simulink model "Basic_DMT"  (R2014b)
settings: Solver=FixedStepDiscrete  SolverMode=SingleTasking  StartTime=0.0  StopTime=25e-6-14e-9*24  RelTol=1e-3
PreLoadFcn:
  | userName = getenv('UserName');
  | 
  | if strcmp(userName,'Tim')
  | cd C:\Users\Tim\Documents\GitHub\MA_1\Basic_DMT
  | else
  | cd C:\Users\Tim-UML\Documents\GitHub\MA_1\Basic_DMT
  | end
InitFcn:
  | userName = getenv('UserName');
  | 
  | if strcmp(userName,'Tim')
  | cd C:\Users\Tim\Documents\GitHub\MA_1\Basic_DMT
  | else
  | cd C:\Users\Tim-UML\Documents\GitHub\MA_1\Basic_DMT
  | end
values from neighbouring files (symbols this model uses):
  a0 = 0.21194908595403703    (= 0.211949085954)    [initScript.m]
  a1 = 0.576101828091926    (= 0.576101828092)    [initScript.m]
  a2 = a0    (= 0.211949085954)    [initScript.m]
  beta = 1    [initScript.m]
  bitPerSymb = 4    [initScript.m]
  chanDownFact = Tchan/SystemPeriod    [initScript.m]
  fftLen = 16    [initScript.m]
  fftLenActive = fftLenDMT    (= 32)    [initScript.m]
  fftLenDMT = 2*fftLen    (= 32)    [initScript.m]
  GI_Active = GI_LenDMT    (= 0)    [initScript.m]
  GI_Len = 0    [initScript.m]
  GI_LenDMT = 0    [initScript.m]
  M = log2(fftLen)    [initScript.m]
  sysgenSystemPeriod = 4e-9    (= 4e-09)    [initScript.m]
  SystemPeriod = 4e-9    (= 4e-09)    [initScript.m]
  upsampleFactor = 1    [initScript.m]
  usedSubCar = 14    [initScript.m]
undefined symbols (not defined in the file or in its folder): bitCount, get, modu_mode, Tb, Ts
libraries: xbsIndex_r4 x822, commdigbbndam3 x59, simulink x42, dspsigops x7, commrandsrc2 x6, dspbuff3 x4, dspxfrm3 x3, dspswit3 x2, commseqgen2 x1, dsparch4 x1, commutil2 x1, dspsnks4 x1
(part 1 of 10)
settings Model: Creator=Tim-UML  LastModifiedBy=Tim-UML
settings DebuggingCC: AssertControl=DisableAll
settings HardwareCC: ProdBitPerLong=64  ProdBitPerPointer=64  ProdWordSize=64  ProdHWDeviceType=Generic->64-bit Embedded Processor (LP64)  TargetHWDeviceType=32-bit Generic

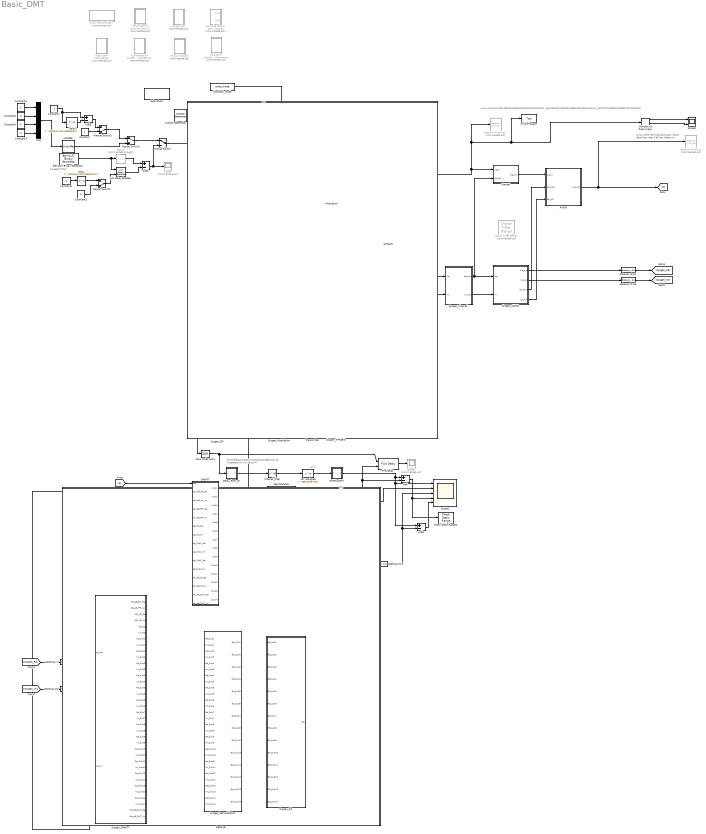
== system Basic_DMT ==
  note: www.marcuswinter.de%2Fmedia%2FOFDM%2FCP%252520spectra.png&imgrefurl=http%3A%2F%2Fwww.marcuswinter.de%2Farchives%2F884&h=684&w=400&tbnid=4qO6ZL-0OhDcYM%3A&docid=MqEDPGI0eCEqiM&ei=dVTEVrCJIeWP6ATR9aGoBQ&tbm=isch&iact=rc&uact=3&dur=395&page=1&start=0&ndsp=36&ved=0ahUKEwjwl_qN1P7KAhXlB5oKHdF6CFUQrQMIIDAA
  note: 477
  note: 1/1.5e8==Ts/3
  note: Umso höher die Modulationsart, desto
      |  deutlicher über 0 dB das Spektrum
  note: 32 singletasking 64 multitasking 256-QAM
      | 16 singletaskink mit 16-QAM
  " System Generator" : xbsIndex_r4/ System Generator  Tag=genX  xilinxfamily=zynq  part=xc7z020  speed=-1  package=clg400  synthesis_tool=Vivado  clock_wrapper=Clock Enables  directory=./netlist  proj_type=Vivado  Synth_file=Vivado Synthesis Defaults  Impl_file=Vivado Implementation Defaults  testbench=off  simulink_period=sysgenSystemPeriod  sysclk_period=1000/250  dcm_input_clock_period=10  incr_netlist=off  trim_vbits=Everywhere in SubSystem  dbl_ovrd=According to Block Masks  core_generation=According to Block Masks  run_coregen=off  deprecated_control=off  eval_field=0  block_type=sysgen
  16-QAM Sysgen : Subsystem  Commented=on
  AWGN : Subsystem  Variant=on
  Add{,1..3} (4 alike) : Sum  Inputs=+-
  Bernoulli Binary Generator : commrandsrc2/Bernoulli Binary Generator  P=0.5  seed=1604198  Ts=Tb  frameBased=off  sampPerFrame=1  orient=off  outDataType=boolean
      settings: AttributesFormatString=|
      | Sample Time= %<Ts>
      | Prob zero=%<P>
  Channel : Subsystem  Variant=on
  Channel_filter : Delay  DelayLength=56  InitialCondition=0
  Check Static Range2 : simulink/Model Verification/Check  Static Range  Description=0 <= u <= 0  max=0  max_included=on  min=0  min_included=on  enabled=off  stopWhenAssertionFail=on  export=off  icon=graphic
  Combination of Sysgen S/P and 16QAM : Subsystem  Commented=on
  Complex to Real-Imag1 : ComplexToRealImag
  Constant : Constant  SampleTime=Tb
  Constant1 : Constant  SampleTime=Tb
  Constant2 : Constant  Value=0  SampleTime=Tb
  Constant3 : Constant  Value=0  SampleTime=Tb*4
  Constant4 : Constant  SampleTime=Tb*4
  Constant5 : Constant  Value=0  SampleTime=Tb*4
  Constant6 : Constant  Value=0  SampleTime=Tb*4
  Constant7 : Constant  SampleTime=Tb
  Constant_mode : Constant  Value=modu_mode  OutDataTypeStr=single
  Delay : Delay  DelayLength=bitPerSymb*usedSubCar-1  InitialCondition=0
  Delay1 : Delay  Commented=through  DelayLength=1  InitialCondition=0
  Delay3 : Delay  DelayLength=bitPerSymb*usedSubCar  InitialCondition=0
  Delay_Rem_GI : Subsystem  Variant=on
  Demodulation : Subsystem
  Digital Filter Design : dsparch4/Digital Filter Design  Commented=on  mwdsp_browser_bugfix_var=off
  Examine Slice Block : Subsystem  Commented=on
  Find Delay : commutil2/Find Delay  corrLength=1000  chgSigOP=off  stopUpdate=off  numConstDelay=3
  Gateway In : xbsIndex_r4/Gateway In  gui_display_data_type=Fixed-point  arith_type="Signed  (2's comp)"  n_bits=bitCount+log2(fftLen)+1  bin_pt=fracLen  preci_type=Single  exp_width=8  frac_width=24  rows=1  columns=1  quantization="Round  (unbiased: +/- Inf)"  overflow=Saturate  period=Ts*M*usedSubCar/(fftLenActive+GI_Active)  UseAsADC=off  ADCChannel='1'  interface=None  automatic_assignment=on  address_offset=hex2dec('00')  intf_description=''  timing_constraint=None  locs_specified=off  LOCs={}  io_standard={}  inherit_from_input=off  hdl_port=on  dbl_ovrd=off  block_type=gatewayin
  Gateway In1 : xbsIndex_r4/Gateway In  gui_display_data_type=Fixed-point  arith_type="Signed  (2's comp)"  n_bits=bitCount+log2(fftLen)+1  bin_pt=fracLen  preci_type=Single  exp_width=8  frac_width=24  rows=1  columns=1  quantization="Round  (unbiased: +/- Inf)"  overflow=Saturate  period=Ts*M*usedSubCar/(fftLenActive+GI_Active)  UseAsADC=off  ADCChannel='1'  interface=None  automatic_assignment=on  address_offset=hex2dec('00')  intf_description=''  timing_constraint=None  locs_specified=off  LOCs={}  io_standard={}  inherit_from_input=off  hdl_port=on  dbl_ovrd=off  block_type=gatewayin
  Gateway Out : xbsIndex_r4/Gateway Out  inherit_from_input=on  hdl_port=on  rows=1  columns=1  UseAsDAC=off  DACChannel='1'  interface=None  automatic_assignment=on  address_offset=hex2dec('00')  intf_description=''  timing_constraint=None  locs_specified=off  LOCs={}  io_standard={}  block_type=gatewayout
  Gateway Out4 : xbsIndex_r4/Gateway Out  inherit_from_input=on  hdl_port=on  rows=1  columns=1  UseAsDAC=off  DACChannel='1'  interface=None  automatic_assignment=on  address_offset=hex2dec('00')  intf_description=''  timing_constraint=None  locs_specified=off  LOCs={}  io_standard={}  block_type=gatewayout
  Gateway Out5 : xbsIndex_r4/Gateway Out  inherit_from_input=on  hdl_port=on  rows=1  columns=1  UseAsDAC=off  DACChannel='1'  interface=None  automatic_assignment=on  address_offset=hex2dec('00')  intf_description=''  timing_constraint=None  locs_specified=off  LOCs={}  io_standard={}  block_type=gatewayout
  IFFTaPIS : Subsystem
  Manual Switch : ManualSwitch
  Manual Switch1 : ManualSwitch
  Manual Switch2 : ManualSwitch  CurrentSetting=0
  Manual Switch3 : ManualSwitch  CurrentSetting=0
  Modulation : Subsystem
  Mux : Mux
  OFDMorDMT : Subsystem  Variant=on
  "PIS " : Subsystem
  Receiver : Subsystem
  "SIP " : Subsystem  RequirementInfo="{}  %GIDa_16a870dd_20fa_4000_a28f_04c7e291452f"
  SIPaFFT : Subsystem
  Scope : Scope  Commented=on
      settings: SaveName=ScopeData65
  Scope1 : Scope  Commented=on
      settings: YMin=-1  YMax=1  SaveName=ScopeData6
  Scope2 : Scope  NumInputPorts=5
      settings: YMin=0~0~0~-1~-1  YMax=1~1~1~1~1  SaveName=ScopeData2
  Scope3 : Scope  NumInputPorts=2
      settings: YMin=-10~-8  YMax=8~8  SaveName=ScopeData30
  Spectrum Analyzer : SpectrumAnalyzer  Commented=on
  Spectrum Analyzer1 : SpectrumAnalyzer  Commented=on
  Subsystem : Subsystem  mask(Model Parameters){upsample=No, dmtOfdm=OFDM, guardInterval=No, AWGN=No, channel=No, equalizer=No, SampleTime=20e-9, BitTime=20e-9, modu_mode=0, radio_precision=double, bitCount=16, fracLen=13, impulseResponse=No}
      mask prompts: upsample "Enable Upsampling"; dmtOfdm "Select FFT Inputorder"; guardInterval "Guard Interval"; SampleTime "Sample Time [s]"; BitTime "Bit Time"; modu_mode "Modulation Mode"; radio_precision "Select Precision"; bitCount "Bit Count"; fracLen "Fraction Length"; impulseResponse "Measure Impulse Response"
      mask init:
      | initScript
      mask TypeOptions upsample: No | Yes
      mask TypeOptions dmtOfdm: OFDM | DMT
      mask TypeOptions guardInterval: No | Yes
      mask TypeOptions AWGN: No | Yes
      mask TypeOptions channel: No | Yes
      mask TypeOptions equalizer: No | Yes
      mask TypeOptions radio_precision: double | fixpoint
      mask TypeOptions impulseResponse: No | Yes
      mask DialogControl Container3 Prompt: Only for Fixpoint
      mask Display: disp('Edit Model\n Parameters')
  Sysgen S/P1 : Subsystem  Commented=on
  Sysgen_AWGN : Subsystem  Variant=on
  Sysgen_Channel : Subsystem  Variant=on
  Sysgen_Demodulation : Subsystem
  Sysgen_IFFTaPIS : Subsystem
  Sysgen_Modulation : Subsystem
  Sysgen_PIS : Subsystem
  Sysgen_SIP : Subsystem
  Sysgen_SIPaFFT : Subsystem
  Testsystem Channelfilter : Subsystem  Commented=on
  Testsystem to examine Demux : Subsystem  Commented=on
  To Workspace : ToWorkspace  VariableName=Test  SampleTime=-1
      settings: Save2DSignal=2-D array (concatenate along first dimension)
  Total Bits / Subchannel Information : Subsystem  Commented=on
  Transmitter : Subsystem
  Unbuffer : Unbuffer  SampleBasedProcessing=Same as frame based
  Unit Delay Enabled : simulink/Additional Math & Discrete/Additional Discrete/Unit Delay Enabled  vinit=0.0  tsamp=-1
  Versuche DEMUX verm. löschen : Subsystem  Commented=on
  Zero-Order Hold : ZeroOrderHold  SampleTime=Ts
  not_assigned : Delay  DelayLength=589-16*8+8*2  InitialCondition=0
  wires:
  Manual Switch/1 -> "SIP "/1(S1), Zero-Order Hold/1, Sysgen_SIP/1(Inp)
  Add/1 -> Scope2/4, Check Static Range2/1
  "PIS "/1(Out) -> Find Delay/2, Add/2, Scope2/2
  Constant_mode/1 -> Demodulation/15(mode), Modulation/15(mode)
  Demodulation/1(Sub1_out) -> "PIS "/1(Sub1)
  Demodulation/2(Sub2_out) -> "PIS "/2(Sub2)
  Modulation/2(Sub2_out) -> IFFTaPIS/2(Sub2)
  SIPaFFT/1(Sub1) -> Demodulation/1(Sub1)
  SIPaFFT/2(Sub2) -> Demodulation/2(Sub2)
  Find Delay/1 -> Scope1/1
  Bernoulli Binary Generator/1 -> Unit Delay Enabled/1, Delay1/1
  Sysgen_Modulation/1(Re_Sub1) -> Modulation/16(db_sub1_re), Sysgen_IFFTaPIS/1(Re_Sub1)
  Modulation/1(Sub1_out) -> IFFTaPIS/1(Sub1)
  "SIP "/2(Sub2) -> Modulation/2(Sub2)
  "SIP "/1(Sub1) -> Modulation/1(Sub1)
  Sysgen_SIP/2(Sub2) -> "SIP "/3(Debug2), Sysgen_Modulation/2(Sub2)
  Sysgen_SIP/1(Sub1) -> "SIP "/2(Debug1), Sysgen_Modulation/1(Sub1)
  Sysgen_IFFTaPIS/1(Re) -> IFFTaPIS/15(db1_aft_GI_Re), Sysgen_Channel/1(Re)
  Gateway Out4/1 -> [Sysgen_Re]
  Gateway Out5/1 -> [Sysgen_Im]
  [A] -> SIPaFFT/1(sig)
  [Sysgen_Re] -> Gateway In/1
  [Sysgen_Im] -> Gateway In1/1
  Gateway In/1 -> Sysgen_SIPaFFT/1(sg_Re), SIPaFFT/2(db_bef_GI_Re)
  Gateway In1/1 -> Sysgen_SIPaFFT/2(sg_Im), SIPaFFT/3(db_bef_GI_Im)
  Sysgen_SIPaFFT/1(db_aft_FFT_Re) -> SIPaFFT/4(db_aft_FFT_Re)
  Sysgen_Demodulation/1(Bit_Sub1) -> Sysgen_PIS/1(Bit_Sub1), Demodulation/16(sg_Sub1_Bit)
  Sysgen_Demodulation/2(Bit_Sub2) -> Sysgen_PIS/2(Bit_Sub2), Demodulation/17(sg_Sub2_Bit)
  Gateway Out/1 -> Scope2/3, Add1/2
  Add1/1 -> Scope2/5
  Sysgen_PIS/1(Bit) -> Gateway Out/1, "PIS "/15(sg_Bit)
  "SIP "/3(Sub3) -> Modulation/3(Sub3)
  "SIP "/4(Sub4) -> Modulation/4(Sub4)
  "SIP "/5(Sub5) -> Modulation/5(Sub5)
  "SIP "/6(Sub6) -> Modulation/6(Sub6)
  "SIP "/7(Sub7) -> Modulation/7(Sub7)
  "SIP "/8(Sub8) -> Modulation/8(Sub8)
  "SIP "/9(Sub9) -> Modulation/9(Sub9)
  "SIP "/10(Sub10) -> Modulation/10(Sub10)
  "SIP "/11(Sub11) -> Modulation/11(Sub11)
  Modulation/3(Sub3_out) -> IFFTaPIS/3(Sub3)
  Modulation/4(Sub4_out) -> IFFTaPIS/4(Sub4)
  Modulation/5(Sub5_out) -> IFFTaPIS/5(Sub5)
  Modulation/6(Sub6_out) -> IFFTaPIS/6(Sub6)
  Modulation/7(Sub7_out) -> IFFTaPIS/7(Sub7)
  Modulation/8(Sub8_out) -> IFFTaPIS/8(Sub8)
  Modulation/9(Sub9_out) -> IFFTaPIS/9(Sub9)
  Modulation/10(Sub10_out) -> IFFTaPIS/10(Sub10)
  Modulation/11(Sub11_out) -> IFFTaPIS/11(Sub11)
  Sysgen_IFFTaPIS/3(Db_aft_frame_Re) -> IFFTaPIS/17(db_aft_frame_Re)
  Sysgen_IFFTaPIS/4(Db_aft_frame_Im) -> IFFTaPIS/18(db_aft_frame_Im)
  Sysgen_IFFTaPIS/5(Db_aft_FFT_Re) -> IFFTaPIS/19(db_FFT_Re)
  Sysgen_IFFTaPIS/6(Db_aft_FFT_Im) -> IFFTaPIS/20(db_FFT_Im)
  SIPaFFT/3(Sub3) -> Demodulation/3(Sub3)
  SIPaFFT/4(Sub4) -> Demodulation/4(Sub4)
  SIPaFFT/5(Sub5) -> Demodulation/5(Sub5)
  SIPaFFT/6(Sub6) -> Demodulation/6(Sub6)
  SIPaFFT/7(Sub7) -> Demodulation/7(Sub7)
  SIPaFFT/8(Sub8) -> Demodulation/8(Sub8)
  SIPaFFT/9(Sub9) -> Demodulation/9(Sub9)
  SIPaFFT/10(Sub10) -> Demodulation/10(Sub10)
  SIPaFFT/11(Sub11) -> Demodulation/11(Sub11)
  Demodulation/3(Sub3_out) -> "PIS "/3(Sub3)
  Demodulation/4(Sub4_out) -> "PIS "/4(Sub4)
  Demodulation/5(Sub5_out) -> "PIS "/5(Sub5)
  Demodulation/6(Sub6_out) -> "PIS "/6(Sub6)
  Demodulation/7(Sub7_out) -> "PIS "/7(Sub7)
  Demodulation/8(Sub8_out) -> "PIS "/8(Sub8)
  Demodulation/9(Sub9_out) -> "PIS "/9(Sub9)
  Demodulation/10(Sub10_out) -> "PIS "/10(Sub10)
  Demodulation/11(Sub11_out) -> "PIS "/11(Sub11)
  Modulation/12(Sub12_out) -> IFFTaPIS/12(Sub12)
  Modulation/13(Sub13_out) -> IFFTaPIS/13(Sub13)
  Modulation/14(Sub14_out) -> IFFTaPIS/14(Sub14)
  SIPaFFT/14(Sub14) -> Demodulation/14(Sub14)
  SIPaFFT/13(Sub13) -> Demodulation/13(Sub13)
  SIPaFFT/12(Sub12) -> Demodulation/12(Sub12)
  Demodulation/13(Sub13_out) -> "PIS "/13(Sub13)
  Demodulation/14(Sub14_out) -> "PIS "/14(Sub14)
  Demodulation/12(Sub12_out) -> "PIS "/12(Sub12)
  "SIP "/12(Sub12) -> Modulation/12(Sub12)
  "SIP "/13(Sub13) -> Modulation/13(Sub13)
  "SIP "/14(Sub14) -> Modulation/14(Sub14)
  OFDMorDMT/1(Out1) -> Add1/1, Scope2/1, Add/1
  Sysgen_SIP/3(Sub3) -> Sysgen_Modulation/3(Sub3)
  Sysgen_SIP/4(Sub4) -> Sysgen_Modulation/4(Sub4)
  Sysgen_SIP/5(Sub5) -> Sysgen_Modulation/5(Sub5)
  Sysgen_SIP/6(Sub6) -> Sysgen_Modulation/6(Sub6)
  Sysgen_SIP/7(Sub7) -> Sysgen_Modulation/7(Sub7)
  Sysgen_SIP/8(Sub8) -> Sysgen_Modulation/8(Sub8)
  Sysgen_SIP/9(Sub9) -> Sysgen_Modulation/9(Sub9)
  Sysgen_SIP/10(Sub10) -> Sysgen_Modulation/10(Sub10)
  Sysgen_SIP/11(Sub11) -> Sysgen_Modulation/11(Sub11)
  Sysgen_SIP/12(Sub12) -> Sysgen_Modulation/12(Sub12)
  Sysgen_SIP/13(Sub13) -> Sysgen_Modulation/13(Sub13)
  Sysgen_SIP/14(Sub14) -> Sysgen_Modulation/14(Sub14)
  Sysgen_Modulation/2(Im_Sub1) -> Modulation/17(db_sub1_im), Sysgen_IFFTaPIS/2(Im_Sub1)
  Sysgen_Modulation/3(Re_Sub2) -> Modulation/18(db_sub2_re), Sysgen_IFFTaPIS/3(Re_Sub2)
  Sysgen_Modulation/4(Im_Sub2) -> Modulation/19(db_sub2_im), Sysgen_IFFTaPIS/4(Im_Sub2)
  Sysgen_Modulation/5(Re_Sub3) -> Sysgen_IFFTaPIS/5(Re_Sub3)
  Sysgen_Modulation/6(Im_Sub3) -> Sysgen_IFFTaPIS/6(Im_Sub3)
  Sysgen_Modulation/7(Re_Sub4) -> Sysgen_IFFTaPIS/7(Re_Sub4)
  Sysgen_Modulation/8(Im_Sub4) -> Sysgen_IFFTaPIS/8(Im_Sub4)
  Sysgen_Modulation/9(Re_Sub5) -> Sysgen_IFFTaPIS/9(Re_Sub5)
  Sysgen_Modulation/10(Im_Sub5) -> Sysgen_IFFTaPIS/10(Im_Sub5)
  Sysgen_Modulation/11(Re_Sub6) -> Sysgen_IFFTaPIS/11(Re_Sub6)
  Sysgen_Modulation/12(Im_Sub6) -> Sysgen_IFFTaPIS/12(Im_Sub6)
  Sysgen_Modulation/13(Re_Sub7) -> Sysgen_IFFTaPIS/13(Re_Sub7)
  Sysgen_Modulation/14(Im_Sub7) -> Sysgen_IFFTaPIS/14(Im_Sub7)
  Sysgen_Modulation/15(Re_Sub8) -> Sysgen_IFFTaPIS/15(Re_Sub8)
  Sysgen_Modulation/16(Im_Sub8) -> Sysgen_IFFTaPIS/16(Im_Sub8)
  Sysgen_Modulation/17(Re_Sub9) -> Sysgen_IFFTaPIS/17(Re_Sub9)
  Sysgen_Modulation/18(Im_Sub9) -> Sysgen_IFFTaPIS/18(Im_Sub9)
  Sysgen_Modulation/19(Re_Sub10) -> Sysgen_IFFTaPIS/19(Re_Sub10)
  Sysgen_Modulation/20(Im_Sub10) -> Sysgen_IFFTaPIS/20(Im_Sub10)
  Sysgen_Modulation/21(Re_Sub11) -> Sysgen_IFFTaPIS/21(Re_Sub11)
  Sysgen_Modulation/22(Im_Sub11) -> Sysgen_IFFTaPIS/22(Im_Sub11)
  Sysgen_Modulation/23(Re_Sub12) -> Sysgen_IFFTaPIS/23(Re_Sub12)
  Sysgen_Modulation/24(Im_Sub12) -> Sysgen_IFFTaPIS/24(Im_Sub12)
  Sysgen_Modulation/25(Re_Sub13) -> Sysgen_IFFTaPIS/25(Re_Sub13)
  Sysgen_Modulation/26(Im_Sub13) -> Sysgen_IFFTaPIS/26(Im_Sub13)
  Sysgen_Modulation/27(Re_Sub14) -> Sysgen_IFFTaPIS/27(Re_Sub14)
  Sysgen_Modulation/28(Im_Sub14) -> Sysgen_IFFTaPIS/28(Im_Sub14)
  not_assigned/1 -> OFDMorDMT/1(In1)
  Sysgen_SIPaFFT/34(Im_Sub14) -> Sysgen_Demodulation/28(Im_Sub14)
  Sysgen_SIPaFFT/33(Re_Sub14) -> Sysgen_Demodulation/27(Re_Sub14)
  Sysgen_SIPaFFT/32(Im_Sub13) -> Sysgen_Demodulation/26(Im_Sub13)
  Sysgen_SIPaFFT/31(Re_Sub13) -> Sysgen_Demodulation/25(Re_Sub13)
  Sysgen_SIPaFFT/30(Im_Sub12) -> Sysgen_Demodulation/24(Im_Sub12)
  Sysgen_SIPaFFT/29(Re_Sub12) -> Sysgen_Demodulation/23(Re_Sub12)
  Sysgen_SIPaFFT/28(Im_Sub11) -> Sysgen_Demodulation/22(Im_Sub11)
  Sysgen_SIPaFFT/27(Re_Sub11) -> Sysgen_Demodulation/21(Re_Sub11)
  Sysgen_SIPaFFT/26(Im_Sub10) -> Sysgen_Demodulation/20(Im_Sub10)
  Sysgen_SIPaFFT/25(Re_Sub10) -> Sysgen_Demodulation/19(Re_Sub10)
  Sysgen_SIPaFFT/24(Im_Sub9) -> Sysgen_Demodulation/18(Im_Sub9)
  Sysgen_SIPaFFT/23(Re_Sub9) -> Sysgen_Demodulation/17(Re_Sub9)
  Sysgen_SIPaFFT/22(Im_Sub8) -> Sysgen_Demodulation/16(Im_Sub8)
  Sysgen_SIPaFFT/21(Re_Sub8) -> Sysgen_Demodulation/15(Re_Sub8)
  Sysgen_SIPaFFT/20(Im_Sub7) -> Sysgen_Demodulation/14(Im_Sub7)
  Sysgen_SIPaFFT/19(Re_Sub7) -> Sysgen_Demodulation/13(Re_Sub7)
  Sysgen_SIPaFFT/18(Im_Sub6) -> Sysgen_Demodulation/12(Im_Sub6)
  Sysgen_SIPaFFT/17(Re_Sub6) -> Sysgen_Demodulation/11(Re_Sub6)
  Sysgen_SIPaFFT/16(Im_Sub5) -> Sysgen_Demodulation/10(Im_Sub5)
  Sysgen_SIPaFFT/15(Re_Sub5) -> Sysgen_Demodulation/9(Re_Sub5)
  Sysgen_SIPaFFT/14(Im_Sub4) -> Sysgen_Demodulation/8(Im_Sub4)
  Sysgen_SIPaFFT/11(Re_Sub3) -> Sysgen_Demodulation/5(Re_Sub3)
  Sysgen_SIPaFFT/12(Im_Sub3) -> Sysgen_Demodulation/6(Im_Sub3)
  Sysgen_SIPaFFT/13(Re_Sub4) -> Sysgen_Demodulation/7(Re_Sub4)
  Sysgen_SIPaFFT/10(Im_Sub2) -> SIPaFFT/11(sg_Sub2_Im), Sysgen_Demodulation/4(Im_Sub2)
  Sysgen_SIPaFFT/9(Re_Sub2) -> SIPaFFT/10(sg_Sub2_Re), Sysgen_Demodulation/3(Re_Sub2)
  Sysgen_SIPaFFT/8(Im_Sub1) -> SIPaFFT/9(sg_Sub1_Im), Sysgen_Demodulation/2(Im_Sub1)
  Sysgen_SIPaFFT/7(Re_Sub1) -> SIPaFFT/8(sg_Sub1_Re), Sysgen_Demodulation/1(Re_Sub1)
  Sysgen_SIPaFFT/2(db_aft_FFT_Im) -> SIPaFFT/5(db_aft_FFT_Im)
  Sysgen_SIPaFFT/3(db2_GI_Re) -> SIPaFFT/12(db_aft_GI_Re)
  Sysgen_SIPaFFT/4(db2_GI_Im) -> SIPaFFT/13(db_aft_GI_Im)
  Sysgen_SIPaFFT/5(Re_DC) -> SIPaFFT/6(sg_DC_Re)
  Sysgen_SIPaFFT/6(Im_DC) -> SIPaFFT/7(sg_DC_Im)
  Sysgen_Demodulation/3(Bit_Sub3) -> Sysgen_PIS/3(Bit_Sub3)
  Sysgen_Demodulation/4(Bit_Sub4) -> Sysgen_PIS/4(Bit_Sub4)
  Sysgen_Demodulation/5(Bit_Sub5) -> Sysgen_PIS/5(Bit_Sub5)
  Sysgen_Demodulation/6(Bit_Sub6) -> Sysgen_PIS/6(Bit_Sub6)
  Sysgen_Demodulation/7(Bit_Sub7) -> Sysgen_PIS/7(Bit_Sub7)
  Sysgen_Demodulation/8(Bit_Sub8) -> Sysgen_PIS/8(Bit_Sub8)
  Sysgen_Demodulation/9(Bit_Sub9) -> Sysgen_PIS/9(Bit_Sub9)
  Sysgen_Demodulation/10(Bit_Sub10) -> Sysgen_PIS/10(Bit_Sub10)
  Sysgen_Demodulation/11(Bit_Sub11) -> Sysgen_PIS/11(Bit_Sub11)
  Sysgen_Demodulation/12(Bit_Sub12) -> Sysgen_PIS/12(Bit_Sub12)
  Sysgen_Demodulation/13(Bit_Sub13) -> Sysgen_PIS/13(Bit_Sub13)
  Sysgen_Demodulation/14(Bit_Sub14) -> Sysgen_PIS/14(Bit_Sub14)
  AWGN/1(sig_out) -> [A], Spectrum Analyzer/1
  Complex to Real-Imag1/1 -> Scope3/1
  Constant/1 -> Manual Switch3/2
  Sysgen_AWGN/1(Re_out) -> Gateway Out4/1
  Sysgen_AWGN/2(Im_out) -> Gateway Out5/1
  Sysgen_AWGN/3(db_bool) -> AWGN/2(db_bool)
  Sysgen_AWGN/4(db_full) -> AWGN/3(db_full)
  Sysgen_IFFTaPIS/2(Im) -> IFFTaPIS/16(db1_aft_GI_Im), Sysgen_Channel/2(Im)
  Sysgen_Channel/1(Re_out) -> Channel/2(db_Re), Sysgen_AWGN/1(Re)
  Sysgen_Channel/2(Im_out) -> Sysgen_AWGN/2(Im)
  Channel_filter/1 -> not_assigned/1
  Channel/1(sig_out) -> AWGN/1(sig_in)
  Sysgen_SIPaFFT/35(db_aft_DMT_Re) -> SIPaFFT/14(db_aft_DMT_Re)
  Sysgen_SIPaFFT/36(db_aft_DMT_Im) -> SIPaFFT/15(db_aft_DMT_Im)
  Delay_Rem_GI/1(Out1) -> Channel_filter/1
  Complex to Real-Imag1/2 -> Scope3/2
  Add2/1 -> Manual Switch/2, Scope/1
  Unit Delay Enabled/1 -> Add2/2
  Delay/1 -> Manual Switch2/1
  Constant1/1 -> Delay/1
  Delay1/1 -> Add2/1
  Manual Switch2/1 -> Unit Delay Enabled/2
  Constant2/1 -> Manual Switch2/2
  Zero-Order Hold/1 -> Delay_Rem_GI/1(In1), Find Delay/1
  Constant3/1 -> Mux/4
  Constant4/1 -> Mux/1
  Constant5/1 -> Mux/2
  Constant6/1 -> Mux/3
  Mux/1 -> Unbuffer/1
  Unbuffer/1 -> Manual Switch1/2
  Manual Switch1/1 -> Manual Switch/1
  Manual Switch3/1 -> Manual Switch1/1
  Add3/1 -> Manual Switch3/1
  Delay3/1 -> Add3/2
  Constant7/1 -> Add3/1, Delay3/1
  IFFTaPIS/1(Out1) -> Channel/1(sig_in), To Workspace/1, Complex to Real-Imag1/1, Spectrum Analyzer1/1

== system Basic_DMT/16-QAM Sysgen ==
  16-QAM : Subsystem
  Check Static Range1 : simulink/Model Verification/Check  Static Range  Description=0 <= u <= 0  max=0  max_included=on  min=0  min_included=on  enabled=on  stopWhenAssertionFail=on  export=off  icon=graphic
  Complex to Real-Imag : ComplexToRealImag
  Constellation Diagram : ConstellationDiagram
  Data Type Conversion : DataTypeConversion  OutDataTypeStr=fixdt(0,4,0)
  Delay : Delay  DelayLength=1  InitialCondition=0
  Gateway In : xbsIndex_r4/Gateway In  gui_display_data_type=Fixed-point  arith_type=Unsigned  n_bits=4  bin_pt=0  preci_type=Single  exp_width=8  frac_width=24  rows=1  columns=1  quantization="Round  (unbiased: +/- Inf)"  overflow=Saturate  period=Tb  UseAsADC=off  ADCChannel='1'  interface=None  automatic_assignment=on  address_offset=hex2dec('00')  intf_description=''  timing_constraint=None  locs_specified=off  LOCs={}  io_standard={}  inherit_from_input=off  hdl_port=on  dbl_ovrd=off  block_type=gatewayin
  Gateway Out : xbsIndex_r4/Gateway Out  inherit_from_input=off  hdl_port=off  rows=1  columns=1  UseAsDAC=off  DACChannel='1'  interface=None  automatic_assignment=on  address_offset=hex2dec('00')  intf_description=''  timing_constraint=None  locs_specified=off  LOCs={}  io_standard={}  block_type=gatewayout
  Gateway Out1 : xbsIndex_r4/Gateway Out  inherit_from_input=off  hdl_port=off  rows=1  columns=1  UseAsDAC=off  DACChannel='1'  interface=None  automatic_assignment=on  address_offset=hex2dec('00')  intf_description=''  timing_constraint=None  locs_specified=off  LOCs={}  io_standard={}  block_type=gatewayout
  Random Integer Generator : commrandsrc2/Random Integer Generator  mul=16  seed=375435435  Ts=Tb  frameBased=off  sampPerFrame=1  orient=off  outDataType=uint8
  Real-Imag to Complex : RealImagToComplex
  Rect_QAM_Mod : commdigbbndam3/Rectangular QAM Modulator Baseband  M=16  InType=Integer  Enc=Gray  Mapping=[0:15]  PowType=Min. distance between symbols  MinDist=2  AvgPow=1  PeakPow=1  Ph=0  outDtype=double  outWordLen=16  outUDDataType=sfix(8)  outFracLenMode=User-defined  outFracLen=0
  Scope1 : Scope  NumInputPorts=4
      settings: YMin=-5~-5~-5~-5  YMax=5~5~5~5
  Scope2 : Scope  NumInputPorts=3
      settings: YMin=-5~-5~-5  YMax=5~5~5  SaveName=ScopeData19
  Scope3 : Scope
      settings: SaveName=ScopeData3
  Subtract : Sum  Inputs=+-
  wires:
  Real-Imag to Complex/1 -> Constellation Diagram/1
  Gateway Out/1 -> Scope2/2, Subtract/2, Real-Imag to Complex/1, Scope1/1
  Gateway Out1/1 -> Real-Imag to Complex/2, Scope1/2
  Gateway In/1 -> 16-QAM/1(In1)
  16-QAM/1(Out2) -> Gateway Out/1
  16-QAM/2(Out3) -> Gateway Out1/1
  Random Integer Generator/1 -> Data Type Conversion/1, Scope3/1, Gateway In/1
  Rect_QAM_Mod/1 -> Delay/1
  Subtract/1 -> Check Static Range1/1, Scope2/3
  Data Type Conversion/1 -> Rect_QAM_Mod/1
  Complex to Real-Imag/1 -> Scope2/1, Subtract/1, Scope1/3
  Delay/1 -> Complex to Real-Imag/1
  Complex to Real-Imag/2 -> Scope1/4

== system Basic_DMT/AWGN ==
  note: 1) Add Subsystem or Model blocks as valid variant choices.
      | 2) You cannot connect blocks at this level. At simulation, connectivity is automatically
      | determined, based on the active variant and port name matching.
  sig_in : Inport
  db_bool : Inport  Port=2
  db_full : Inport  Port=3
  No_AWGN : Subsystem  VariantControl=AWGN==1
  Yes_AWGN : Subsystem  VariantControl=AWGN==2
  sig_out : Outport

== system Basic_DMT/Channel ==
  note: 1) Add Subsystem or Model blocks as valid variant choices.
      | 2) You cannot connect blocks at this level. At simulation, connectivity is automatically
      | determined, based on the active variant and port name matching.
  sig_in : Inport
  db_Re : Inport  Port=2
  No_channel : Subsystem  VariantControl=channel==1
  Yes_Channel : Subsystem  VariantControl=channel==2
  sig_out : Outport

== system Basic_DMT/Combination of Sysgen S//P and 16QAM ==
  note: Fehlerhaft, also muss das Problem in der Zuführung der BIts in den Simulink QAM Block liegen
      | Oder im Sysgen Serial to Parallel Endianness
  note: FUnktioniert Fehlerfrei
  16-QAM 1 : Subsystem
  16-QAM 2 : Subsystem
  Bernoulli Binary Generator1 : commrandsrc2/Bernoulli Binary Generator  P=0.5  seed=1604198  Ts=Tb  frameBased=off  sampPerFrame=1  orient=off  outDataType=boolean
      settings: AttributesFormatString=|
      | Sample Time= %<Ts>
      | Prob zero=%<P>
  BitBasher : xbsIndex_r4/BitBasher  bitexpr=|  display_expr=on  sr_1=y1  arith_type1=Unsigned  bin_pt1=0  sr_2=y2  arith_type2=Unsigned  bin_pt2=0  sr_3=3  arith_type3=Unsigned  bin_pt3=0  sr_4=4  arith_type4=Unsigned  bin_pt4=0  dbl_ovrd=off  block_type=bitbasher
      | y1={a[7:4]}
      | y2={a[3:0]}
  Buffer : Buffer  N=8  TreatMby1Signals=One channel
  Check Static Range{1..4} (4 alike) : simulink/Model Verification/Check  Static Range  Description=0 <= u <= 0  max=0  max_included=on  min=0  min_included=on  enabled=on  stopWhenAssertionFail=on  export=off  icon=graphic
  Complex to Real-Imag1 : ComplexToRealImag
  Complex to Real-Imag2 : ComplexToRealImag
  Constellation Diagram2 : ConstellationDiagram
  Counter Limited2 : simulink/Sources/Counter Limited  uplimit=1  tsamp=Tb
  Delay1 : Delay  DelayLength=1  InitialCondition=0  InputProcessing=Columns as channels (frame based)
  Delay2 : Delay  DelayLength=1  InitialCondition=0
  Delay3 : Delay  DelayLength=1  InitialCondition=0
  Delay4 : Delay  DelayLength=1  InitialCondition=0
  Demux : Demux  Outputs=2
  Gateway In1 : xbsIndex_r4/Gateway In  gui_display_data_type=Fixed-point  arith_type=Unsigned  n_bits=1  bin_pt=0  preci_type=Single  exp_width=8  frac_width=24  rows=1  columns=1  quantization="Round  (unbiased: +/- Inf)"  overflow=Saturate  period=Ts  UseAsADC=off  ADCChannel='1'  interface=None  automatic_assignment=on  address_offset=hex2dec('00')  intf_description=''  timing_constraint=None  locs_specified=off  LOCs={}  io_standard={}  inherit_from_input=off  hdl_port=on  dbl_ovrd=off  block_type=gatewayin
  Gateway Out : xbsIndex_r4/Gateway Out  inherit_from_input=on  hdl_port=off  rows=1  columns=1  UseAsDAC=off  DACChannel='1'  interface=None  automatic_assignment=on  address_offset=hex2dec('00')  intf_description=''  timing_constraint=None  locs_specified=off  LOCs={}  io_standard={}  block_type=gatewayout
  Gateway Out1 : xbsIndex_r4/Gateway Out  inherit_from_input=on  hdl_port=off  rows=1  columns=1  UseAsDAC=off  DACChannel='1'  interface=None  automatic_assignment=on  address_offset=hex2dec('00')  intf_description=''  timing_constraint=None  locs_specified=off  LOCs={}  io_standard={}  block_type=gatewayout
  Gateway Out{2..5} (4 alike) : xbsIndex_r4/Gateway Out  inherit_from_input=off  hdl_port=off  rows=1  columns=1  UseAsDAC=off  DACChannel='1'  interface=None  automatic_assignment=on  address_offset=hex2dec('00')  intf_description=''  timing_constraint=None  locs_specified=off  LOCs={}  io_standard={}  block_type=gatewayout
  Gateway Out8 : xbsIndex_r4/Gateway Out  inherit_from_input=on  hdl_port=off  rows=1  columns=1  UseAsDAC=off  DACChannel='1'  interface=None  automatic_assignment=on  address_offset=hex2dec('00')  intf_description=''  timing_constraint=None  locs_specified=off  LOCs={}  io_standard={}  block_type=gatewayout
  Manual Switch1 : ManualSwitch  CurrentSetting=0
  Parallel to Serial : xbsIndex_r4/Parallel to Serial  output_order=Most Significant Word First  arith_type=Unsigned  output_bits=1  bin_pt=0  rst=off  en=off  latency=1  dbl_ovrd=off  block_type=p2s
      settings: infoedit=Each sample presented at the input becomes several samples presented serially at the output.
  Parallel to Serial1 : xbsIndex_r4/Parallel to Serial  output_order=Most Significant Word First  arith_type=Unsigned  output_bits=1  bin_pt=0  rst=off  en=off  latency=1  dbl_ovrd=off  block_type=p2s
      settings: infoedit=Each sample presented at the input becomes several samples presented serially at the output.
  Real-Imag to Complex2 : RealImagToComplex
  Rect_QAM_Mod : commdigbbndam3/Rectangular QAM Modulator Baseband  M=16  InType=Integer  Enc=Gray  Mapping=[0:15]  PowType=Min. distance between symbols  MinDist=2  AvgPow=1  PeakPow=1  Ph=0  outDtype=double  outWordLen=16  outUDDataType=sfix(8)  outFracLenMode=User-defined  outFracLen=0
  Rect_QAM_Mod1 : commdigbbndam3/Rectangular QAM Modulator Baseband  M=16  InType=Bit  Enc=Gray  Mapping=[0:15]  PowType=Min. distance between symbols  MinDist=2  AvgPow=1  PeakPow=1  Ph=0  outDtype=double  outWordLen=16  outUDDataType=sfix(8)  outFracLenMode=User-defined  outFracLen=0
  Scope2 : Scope  NumInputPorts=3
      settings: YMin=-5~-5~-5  YMax=5~5~5  SaveName=ScopeData17
  Scope3 : Scope  NumInputPorts=4
      settings: YMin=-5~-5~-5~-5  YMax=5~5~5~5  SaveName=ScopeData9
  Scope5 : Scope  NumInputPorts=4
      settings: YMin=-5~-5~-5~-5  YMax=5~5~5~5  SaveName=ScopeData10
  Scope6 : Scope  NumInputPorts=3
      settings: YMin=-5~-5~-5  YMax=5~5~5  SaveName=ScopeData12
  Serial to Parallel : xbsIndex_r4/Serial to Parallel  input_order=Most Significant Word First  arith_type=Unsigned  output_bits=8  bin_pt=0  rst=off  en=off  latency=1  dbl_ovrd=off  block_type=s2p
      settings: infoedit=Groups of samples presented serially at the input become single samples presented at the output.
  Subtract{,1..3} (4 alike) : Sum  Inputs=+-
  Terminator : Terminator
  Terminator1 : Terminator
  Unbuffer : Unbuffer  SampleBasedProcessing=Same as frame based
  Unbuffer1 : Unbuffer  SampleBasedProcessing=Same as frame based
  wires:
  Subtract1/1 -> Check Static Range4/1, Scope3/4
  Gateway Out1/1 -> Scope3/2, Subtract1/2
  Bernoulli Binary Generator1/1 -> Manual Switch1/2
  Demux/1 -> Rect_QAM_Mod1/1, Unbuffer1/1
  Manual Switch1/1 -> Buffer/1, Gateway In1/1
  Parallel to Serial/1 -> Gateway Out/1
  Buffer/1 -> Demux/1
  Gateway In1/1 -> Serial to Parallel/1
  Demux/2 -> Unbuffer/1
  Unbuffer/1 -> Delay3/1
  Serial to Parallel/1 -> BitBasher/1
  Parallel to Serial1/1 -> Gateway Out1/1
  Subtract/1 -> Check Static Range3/1, Scope3/3
  Delay3/1 -> Subtract1/1
  BitBasher/2 -> Parallel to Serial1/1
  Counter Limited2/1 -> Manual Switch1/1
  Gateway Out/1 -> Scope3/1, Subtract/2
  Delay2/1 -> Subtract/1
  Real-Imag to Complex2/1 -> Constellation Diagram2/1
  Gateway Out2/1 -> Scope6/2, Subtract2/2, Scope5/1, Real-Imag to Complex2/1
  Gateway Out3/1 -> Real-Imag to Complex2/2, Scope5/2
  16-QAM 2/1(Out2) -> Gateway Out2/1
  Gateway Out8/1 -> Rect_QAM_Mod/1
  Complex to Real-Imag1/1 -> Scope5/3, Scope6/1, Subtract2/1
  Delay4/1 -> Complex to Real-Imag1/1
  Complex to Real-Imag1/2 -> Scope5/4
  16-QAM 2/2(Out3) -> Gateway Out3/1
  Rect_QAM_Mod/1 -> Delay4/1
  Subtract2/1 -> Check Static Range2/1, Scope6/3
  Gateway Out4/1 -> Scope2/2, Subtract3/2
  16-QAM 1/1(Out2) -> Gateway Out4/1
  Unbuffer1/1 -> Delay2/1
  Complex to Real-Imag2/1 -> Scope2/1, Subtract3/1
  Delay1/1 -> Complex to Real-Imag2/1
  BitBasher/1 -> Gateway Out8/1, 16-QAM 1/1(In1), 16-QAM 2/1(In1), Parallel to Serial/1
  16-QAM 1/2(Out3) -> Gateway Out5/1
  Rect_QAM_Mod1/1 -> Delay1/1
  Subtract3/1 -> Check Static Range1/1, Scope2/3
  Gateway Out5/1 -> Terminator/1
  Complex to Real-Imag2/2 -> Terminator1/1

== system Basic_DMT/Delay_Rem_GI ==
  note: 1) Add Subsystem or Model blocks as valid variant choices.
      | 2) You cannot connect blocks at this level. At simulation, connectivity is automatically
      | determined, based on the active variant and port name matching.
  In1 : Inport
  Delay_GI_DMT : Subsystem  VariantControl=guardInterval==2&&dmtOfdm==2
  Delay_GI_OFDM : Subsystem  VariantControl=guardInterval==2&&dmtOfdm==1
  Delay_None : Subsystem  VariantControl=guardInterval==1
  Out1 : Outport

== system Basic_DMT/Demodulation ==
  Sub1 : Inport
  Sub2 : Inport  Port=2
  Sub3 : Inport  Port=3
  Sub4 : Inport  Port=4
  Sub5 : Inport  Port=5
  Sub6 : Inport  Port=6
  Sub7 : Inport  Port=7
  Sub8 : Inport  Port=8
  Sub9 : Inport  Port=9
  Sub10 : Inport  Port=10
  Sub11 : Inport  Port=11
  Sub12 : Inport  Port=12
  Sub13 : Inport  Port=13
  Sub14 : Inport  Port=14
  mode : Inport  Port=15
  sg_Sub1_Bit : Inport  Port=16
  sg_Sub2_Bit : Inport  Port=17
  Assert_Bit_Mapping : Subsystem
  Bit Demapping P1 : Subsystem
  Bit Demapping P10 : Subsystem
  Bit Demapping P11 : Subsystem
  Bit Demapping P12 : Subsystem
  Bit Demapping P13 : Subsystem
  Bit Demapping P14 : Subsystem
  Bit Demapping P2 : Subsystem
  Bit Demapping P3 : Subsystem
  Bit Demapping P4 : Subsystem
  Bit Demapping P5 : Subsystem
  Bit Demapping P6 : Subsystem
  Bit Demapping P7 : Subsystem
  Bit Demapping P8 : Subsystem
  Bit Demapping P9 : Subsystem
  Delay2 : Delay  Commented=through  DelayLength=1  InitialCondition=0
  Delay3 : Delay  Commented=through  DelayLength=1  InitialCondition=0
  Sub1_out : Outport
  Sub2_out : Outport  Port=2
  Sub3_out : Outport  Port=3
  Sub4_out : Outport  Port=4
  Sub5_out : Outport  Port=5
  Sub6_out : Outport  Port=6
  Sub7_out : Outport  Port=7
  Sub8_out : Outport  Port=8
  Sub9_out : Outport  Port=9
  Sub10_out : Outport  Port=10
  Sub11_out : Outport  Port=11
  Sub12_out : Outport  Port=12
  Sub13_out : Outport  Port=13
  Sub14_out : Outport  Port=14
  wires:
  Sub1/1 -> Bit Demapping P1/2(data)
  Sub2/1 -> Bit Demapping P2/2(data)
  Bit Demapping P1/1(Out1) -> Delay2/1
  Bit Demapping P2/1(Out1) -> Delay3/1
  Delay2/1 -> Assert_Bit_Mapping/1(In1), Sub1_out/1
  Delay3/1 -> Assert_Bit_Mapping/2(In2), Sub2_out/1
  sg_Sub1_Bit/1 -> Assert_Bit_Mapping/3(In3)
  Sub3/1 -> Bit Demapping P3/2(data)
  Bit Demapping P3/1(Out1) -> Sub3_out/1
  Sub4/1 -> Bit Demapping P4/2(data)
  Bit Demapping P4/1(Out1) -> Sub4_out/1
  Sub5/1 -> Bit Demapping P5/2(data)
  Bit Demapping P5/1(Out1) -> Sub5_out/1
  Sub6/1 -> Bit Demapping P6/2(data)
  Bit Demapping P6/1(Out1) -> Sub6_out/1
  Sub7/1 -> Bit Demapping P7/2(data)
  Bit Demapping P7/1(Out1) -> Sub7_out/1
  Sub8/1 -> Bit Demapping P8/2(data)
  Bit Demapping P8/1(Out1) -> Sub8_out/1
  Sub9/1 -> Bit Demapping P9/2(data)
  Bit Demapping P9/1(Out1) -> Sub9_out/1
  Sub10/1 -> Bit Demapping P10/2(data)
  Bit Demapping P10/1(Out1) -> Sub10_out/1
  Sub11/1 -> Bit Demapping P11/2(data)
  Bit Demapping P11/1(Out1) -> Sub11_out/1
  sg_Sub2_Bit/1 -> Assert_Bit_Mapping/4(In4)
  Sub12/1 -> Bit Demapping P14/2(data)
  Bit Demapping P14/1(Out1) -> Sub12_out/1
  Sub13/1 -> Bit Demapping P12/2(data)
  Bit Demapping P12/1(Out1) -> Sub13_out/1
  Sub14/1 -> Bit Demapping P13/2(data)
  Bit Demapping P13/1(Out1) -> Sub14_out/1
  mode/1 -> Bit Demapping P10/1(mode), Bit Demapping P14/1(mode), Bit Demapping P12/1(mode), Bit Demapping P13/1(mode), Bit Demapping P11/1(mode), Bit Demapping P9/1(mode), Bit Demapping P8/1(mode), Bit Demapping P7/1(mode), Bit Demapping P6/1(mode), Bit Demapping P5/1(mode), Bit Demapping P4/1(mode), Bit Demapping P3/1(mode), Bit Demapping P2/1(mode), Bit Demapping P1/1(mode)

== system Basic_DMT/Examine Slice Block ==
  Counter Limited1 : simulink/Sources/Counter Limited  uplimit=255  tsamp=Tb*8
  Counter Limited2 : simulink/Sources/Counter Limited  uplimit=1  tsamp=Tb
  Gateway In : xbsIndex_r4/Gateway In  gui_display_data_type=Fixed-point  arith_type=Unsigned  n_bits=8  bin_pt=0  preci_type=Single  exp_width=8  frac_width=24  rows=1  columns=1  quantization="Round  (unbiased: +/- Inf)"  overflow=Saturate  period=Ts*8  UseAsADC=off  ADCChannel='1'  interface=None  automatic_assignment=on  address_offset=hex2dec('00')  intf_description=''  timing_constraint=None  locs_specified=off  LOCs={}  io_standard={}  inherit_from_input=off  hdl_port=on  dbl_ovrd=off  block_type=gatewayin
  Gateway In1 : xbsIndex_r4/Gateway In  gui_display_data_type=Fixed-point  arith_type=Unsigned  n_bits=1  bin_pt=0  preci_type=Single  exp_width=8  frac_width=24  rows=1  columns=1  quantization="Round  (unbiased: +/- Inf)"  overflow=Saturate  period=Ts  UseAsADC=off  ADCChannel='1'  interface=None  automatic_assignment=on  address_offset=hex2dec('00')  intf_description=''  timing_constraint=None  locs_specified=off  LOCs={}  io_standard={}  inherit_from_input=off  hdl_port=on  dbl_ovrd=off  block_type=gatewayin
  Gateway Out{,1..5} (6 alike) : xbsIndex_r4/Gateway Out  inherit_from_input=on  hdl_port=off  rows=1  columns=1  UseAsDAC=off  DACChannel='1'  interface=None  automatic_assignment=on  address_offset=hex2dec('00')  intf_description=''  timing_constraint=None  locs_specified=off  LOCs={}  io_standard={}  block_type=gatewayout
  Scope : Scope  NumInputPorts=3
      settings: YMin=-5~-5~-5  YMax=5~5~5  SaveName=ScopeData13
  Scope1 : Scope  NumInputPorts=4
      settings: YMin=-5~-5~-5~-5  YMax=5~5~5~5  SaveName=ScopeData22
  Serial to Parallel : xbsIndex_r4/Serial to Parallel  input_order=Most Significant Word First  arith_type=Unsigned  output_bits=8  bin_pt=0  rst=off  en=off  latency=1  dbl_ovrd=off  block_type=s2p
      settings: infoedit=Groups of samples presented serially at the input become single samples presented at the output.
  Slice : xbsIndex_r4/Slice  nbits=4  boolean_output=off  mode=Lower Bit Location + Width  bit1=0  base1=MSB of Input  bit0=0  base0=LSB of Input  dbl_ovrd=off  block_type=slice
  Slice1 : xbsIndex_r4/Slice  nbits=4  boolean_output=off  mode=Lower Bit Location + Width  bit1=0  base1=MSB of Input  bit0=4  base0=LSB of Input  dbl_ovrd=off  block_type=slice
  Slice2 : xbsIndex_r4/Slice  nbits=4  boolean_output=off  mode=Lower Bit Location + Width  bit1=0  base1=MSB of Input  bit0=0  base0=LSB of Input  dbl_ovrd=off  block_type=slice
  Slice3 : xbsIndex_r4/Slice  nbits=4  boolean_output=off  mode=Lower Bit Location + Width  bit1=0  base1=MSB of Input  bit0=4  base0=LSB of Input  dbl_ovrd=off  block_type=slice
  no difference : xbsIndex_r4/Reinterpret  Commented=through  force_arith_type=on  arith_type="Signed  (2's comp)"  force_bin_pt=on  bin_pt=4  block_type=reinterpret
  no difference1 : xbsIndex_r4/Reinterpret  force_arith_type=on  arith_type=Unsigned  force_bin_pt=off  bin_pt=4  block_type=reinterpret
  wires:
  Gateway In/1 -> no difference/1
  Slice/1 -> Gateway Out/1
  Counter Limited1/1 -> Scope/1, Gateway In/1
  Gateway Out/1 -> Scope/2
  Slice1/1 -> Gateway Out1/1
  Gateway Out1/1 -> Scope/3
  no difference/1 -> Slice1/1, Slice/1
  Gateway In1/1 -> Gateway Out5/1, Serial to Parallel/1
  Slice2/1 -> Gateway Out2/1
  Counter Limited2/1 -> Gateway In1/1
  Gateway Out2/1 -> Scope1/2
  Slice3/1 -> Gateway Out3/1
  Gateway Out3/1 -> Scope1/3
  Gateway Out4/1 -> Scope1/1
  Serial to Parallel/1 -> no difference1/1, Slice3/1, Slice2/1
  no difference1/1 -> Gateway Out4/1
  Gateway Out5/1 -> Scope1/4

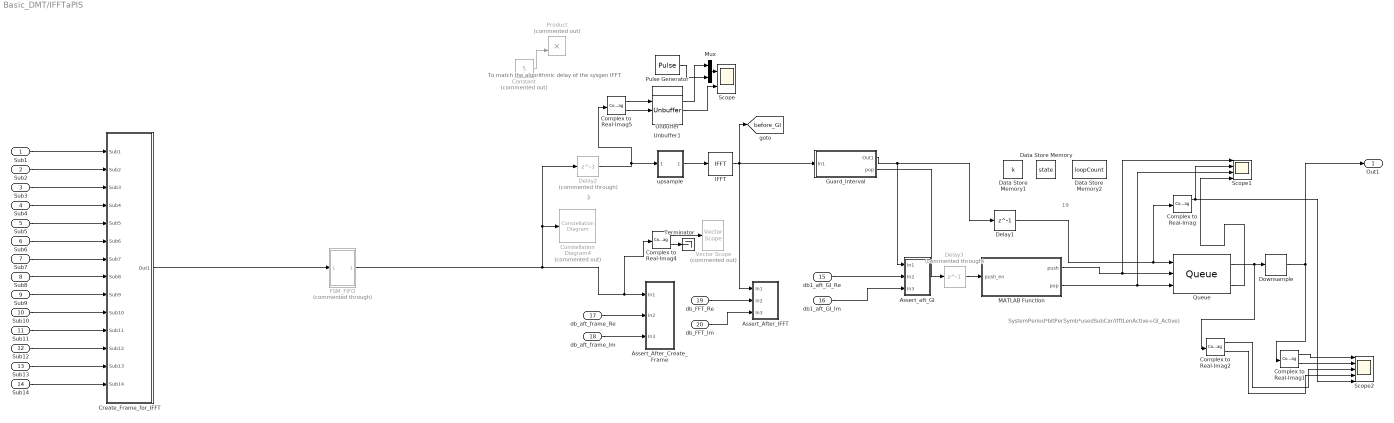
== system Basic_DMT/IFFTaPIS ==
  note: SystemPeriod*bitPerSymb*usedSubCar/(fftLenActive+GI_Active)
  note: 19
  note: 3
  note: To match the algorithmic delay of the sysgen IFFT
  Sub1 : Inport
  Sub2 : Inport  Port=2
  Sub3 : Inport  Port=3
  Sub4 : Inport  Port=4
  Sub5 : Inport  Port=5
  Sub6 : Inport  Port=6
  Sub7 : Inport  Port=7
  Sub8 : Inport  Port=8
  Sub9 : Inport  Port=9
  Sub10 : Inport  Port=10
  Sub11 : Inport  Port=11
  Sub12 : Inport  Port=12
  Sub13 : Inport  Port=13
  Sub14 : Inport  Port=14
  db1_aft_GI_Re : Inport  Port=15
  db1_aft_GI_Im : Inport  Port=16
  db_aft_frame_Re : Inport  Port=17
  db_aft_frame_Im : Inport  Port=18
  db_FFT_Re : Inport  Port=19
  db_FFT_Im : Inport  Port=20
  Assert_After_Create_Frame : Subsystem
  Assert_After_IFFT : Subsystem
  Assert_aft_GI : Subsystem
  Complex to Real-Imag{,1..2,4..5} (5 alike) : ComplexToRealImag
  Constant : Constant  Commented=on  Value=5
  Constellation Diagram4 : ConstellationDiagram  Commented=on
  Create_Frame_for_IFFT : Subsystem
  Data Store Memory : DataStoreMemory  DataStoreName=state  OutDataTypeStr=double
  Data Store Memory1 : DataStoreMemory  DataStoreName=k  OutDataTypeStr=double
  Data Store Memory2 : DataStoreMemory  DataStoreName=loopCount  OutDataTypeStr=double
  Delay1 : Delay  DelayLength=1  InitialCondition=0
  Delay2 : Delay  Commented=through  DelayLength=3  InitialCondition=0
  Delay3 : Delay  Commented=through  DelayLength=1  InitialCondition=0
  Downsample : dspsigops/Downsample  N=chanDownFact  phase=0  RateOptions=Allow multirate processing  smode=Allow multirate  fmode=Maintain input frame size  ic=0
  FSM_FIFO : Subsystem  Commented=through
  Guard_Interval : Subsystem  Variant=on
  IFFT : dspxfrm3/IFFT  CompMethod=Table lookup  TableOpt=NEW  TableOptActive=Speed  BitRevOrder=off  cs_in=off  SkipNorm=off  InheritFFTLength=on  FFTLength=64  WrapInput=on  mode=Complex  outSamplingMode=Sample based  RowConvenienceOn=on  FFTImplementation=Auto  firstCoeffDataTypeStr=Inherit: Same word length as input  firstCoeffLastDataTypeStr=Inherit: Same word length as input  outputMin=[]  outputMax=[]  roundingMode=Convergent  overflowMode=on
  MATLAB Function : MATLAB Function  TreatAsAtomicUnit=on  SystemSampleTime=SystemPeriod*bitPerSymb*usedSubCar/fftLenActive
  Mux : Mux  Inputs=2
  Product : Product  Commented=on  RndMeth=Convergent  SaturateOnIntegerOverflow=on
  Pulse Generator : DiscretePulseGenerator  Amplitude=0.5  Period=fftLenActive*2  PulseWidth=fftLenActive  SampleTime=SystemPeriod*bitPerSymb*usedSubCar/(fftLenActive)
  Queue : dspbuff3/Queue  depth=64  trigger=Non-zero sample  overflow=Dynamic reallocation  pes=Warning  eso=off  fso=off  nso=on  clr=off  clrOutport=off  adf=off
  Scope : Scope  NumInputPorts=2
      settings: YMin=-5~-5  YMax=5~5  SaveName=ScopeData68
  Scope1 : Scope  NumInputPorts=4
      settings: YMin=0~-100~0~0  YMax=1~100~1~30  SaveName=ScopeData72
  Scope2 : Scope  NumInputPorts=5
      settings: YMin=-100~-1~-100~-5~-5  YMax=80~1~80~5~5  SaveName=ScopeData74
  Terminator : Terminator
  Unbuffer : Unbuffer  SampleBasedProcessing=Same as frame based
  Unbuffer1 : Unbuffer  SampleBasedProcessing=Same as frame based
  Vector Scope : dspsnks4/Vector Scope  Commented=on  ScopeProperties=on  Domain=Time  HorizSpan=1000  DisplayProperties=off  AxisGrid=on  Memory=off  FrameNumber=on  AxisLegend=off  AxisZoom=off  OpenScopeAtSimStart=on  OpenScopeImmediately=off  FigPos=get(0,'defaultfigureposition')  AxisProperties=off  XUnits=Hertz  XRange=[0...Fs/2]  InheritXIncr=on  XIncr=1  XLabel=Time  XLimit=Auto  XMin=0  XMax=1  XStart=0  YUnits=dB  YLabel=Amplitude  LineProperties=off  LineMarkers=x  XAxisParamsVer=6.9
      settings: YMin=-10  YMax=10
  upsample : Subsystem  Variant=on
  Out1 : Outport
  tag scope: before_GI=global
  wires:
  Sub1/1 -> Create_Frame_for_IFFT/1(Sub1)
  Sub2/1 -> Create_Frame_for_IFFT/2(Sub2)
  db1_aft_GI_Re/1 -> Assert_aft_GI/2(In2)
  db1_aft_GI_Im/1 -> Assert_aft_GI/3(In3)
  db_aft_frame_Re/1 -> Assert_After_Create_Frame/2(In2)
  db_aft_frame_Im/1 -> Assert_After_Create_Frame/3(In3)
  Delay2/1 -> Complex to Real-Imag5/1, upsample/1(In1)
  IFFT/1 -> Assert_After_IFFT/1(In1), Guard_Interval/1(In1), [before_GI]
  db_FFT_Im/1 -> Assert_After_IFFT/3(In3)
  db_FFT_Re/1 -> Assert_After_IFFT/2(In2)
  Sub3/1 -> Create_Frame_for_IFFT/3(Sub3)
  Sub4/1 -> Create_Frame_for_IFFT/4(Sub4)
  Sub5/1 -> Create_Frame_for_IFFT/5(Sub5)
  Sub6/1 -> Create_Frame_for_IFFT/6(Sub6)
  Sub7/1 -> Create_Frame_for_IFFT/7(Sub7)
  Sub8/1 -> Create_Frame_for_IFFT/8(Sub8)
  Sub9/1 -> Create_Frame_for_IFFT/9(Sub9)
  Sub10/1 -> Create_Frame_for_IFFT/10(Sub10)
  Sub11/1 -> Create_Frame_for_IFFT/11(Sub11)
  Sub13/1 -> Create_Frame_for_IFFT/13(Sub13)
  Sub14/1 -> Create_Frame_for_IFFT/14(Sub14)
  Sub12/1 -> Create_Frame_for_IFFT/12(Sub12)
  upsample/1(Out1) -> IFFT/1
  Constant/1 -> Product/2
  Guard_Interval/1(Out1) -> Delay1/1, Assert_aft_GI/1(In1)
  MATLAB Function/2(pop) -> Scope1/3, Queue/3
  Queue/2 -> Scope1/4
  Complex to Real-Imag1/1 -> Scope2/1
  Complex to Real-Imag1/2 -> Scope2/2
  Complex to Real-Imag/1 -> Scope1/2, Scope2/5
  Queue/1 -> Complex to Real-Imag2/1, Downsample/1
  Downsample/1 -> Out1/1, Complex to Real-Imag1/1
  Complex to Real-Imag2/1 -> Scope2/3
  Complex to Real-Imag2/2 -> Scope2/4
  Complex to Real-Imag4/1 -> Vector Scope/1
  MATLAB Function/1(push) -> Scope1/1, Queue/2
  Mux/1 -> Scope/1
  Complex to Real-Imag5/1 -> Unbuffer/1
  Complex to Real-Imag4/2 -> Terminator/1
  Complex to Real-Imag5/2 -> Unbuffer1/1
  Delay1/1 -> Complex to Real-Imag/1, Queue/1
  Guard_Interval/2(pop) -> Delay3/1
  Delay3/1 -> MATLAB Function/1(push_en)
  FSM_FIFO/1(Out1) -> Delay2/1, Constellation Diagram4/1, Complex to Real-Imag4/1, Assert_After_Create_Frame/1(In1)
  Unbuffer1/1 -> Scope/2
  Unbuffer/1 -> Mux/1
  Pulse Generator/1 -> Mux/2
  Create_Frame_for_IFFT/1(Out1) -> FSM_FIFO/1(In1)

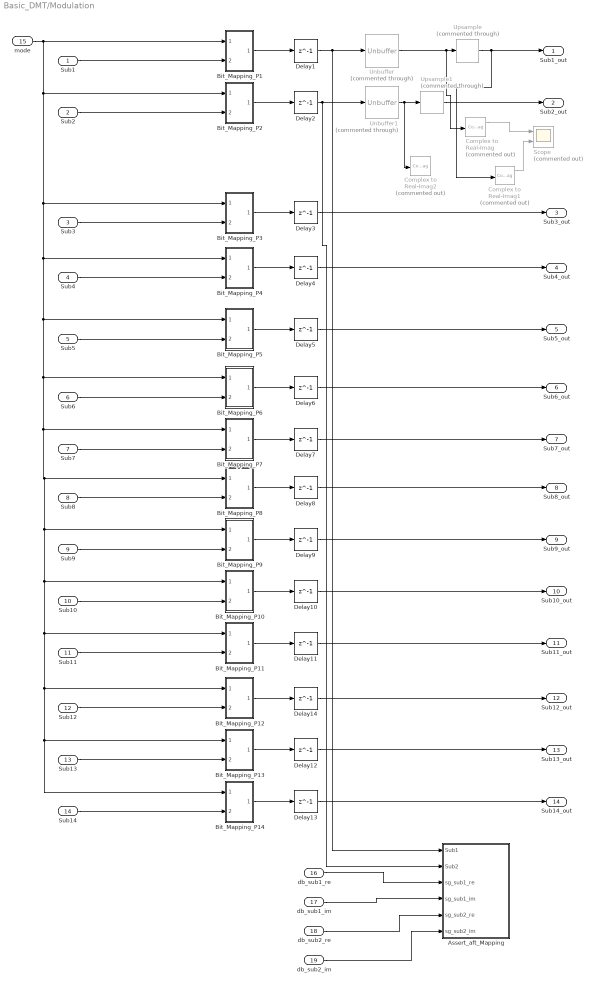
== system Basic_DMT/Modulation ==
  Sub1 : Inport
  Sub2 : Inport  Port=2
  Sub3 : Inport  Port=3
  Sub4 : Inport  Port=4
  Sub5 : Inport  Port=5
  Sub6 : Inport  Port=6
  Sub7 : Inport  Port=7
  Sub8 : Inport  Port=8
  Sub9 : Inport  Port=9
  Sub10 : Inport  Port=10
  Sub11 : Inport  Port=11
  Sub12 : Inport  Port=12
  Sub13 : Inport  Port=13
  Sub14 : Inport  Port=14
  mode : Inport  Port=15
  db_sub1_re : Inport  Port=16
  db_sub1_im : Inport  Port=17
  db_sub2_re : Inport  Port=18
  db_sub2_im : Inport  Port=19
  Assert_aft_Mapping : Subsystem
  Bit_Mapping_P1 : Subsystem
  Bit_Mapping_P10 : Subsystem
  Bit_Mapping_P11 : Subsystem
  Bit_Mapping_P12 : Subsystem
  Bit_Mapping_P13 : Subsystem
  Bit_Mapping_P14 : Subsystem
  Bit_Mapping_P2 : Subsystem
  Bit_Mapping_P3 : Subsystem
  Bit_Mapping_P4 : Subsystem
  Bit_Mapping_P5 : Subsystem
  Bit_Mapping_P6 : Subsystem
  Bit_Mapping_P7 : Subsystem
  Bit_Mapping_P8 : Subsystem
  Bit_Mapping_P9 : Subsystem
  Complex to Real-Imag : ComplexToRealImag  Commented=on
  Complex to Real-Imag1 : ComplexToRealImag  Commented=on
  Complex to Real-Imag2 : ComplexToRealImag  Commented=on
  Delay{1..14} (14 alike) : Delay  DelayLength=1  InitialCondition=0  InputProcessing=Columns as channels (frame based)
  Scope : Scope  Commented=on  NumInputPorts=2
      settings: YMin=-5~-5  YMax=5~5  SaveName=ScopeData45
  Unbuffer : Unbuffer  Commented=through  SampleBasedProcessing=Same as frame based
  Unbuffer1 : Unbuffer  Commented=through  SampleBasedProcessing=Same as frame based
  Upsample : dspsigops/Upsample  Commented=through  N=5  phase=0  RateOptions=Allow multirate processing  ic=0  mode=Unused parameter value
  Upsample1 : dspsigops/Upsample  Commented=through  N=5  phase=0  RateOptions=Allow multirate processing  ic=0  mode=Unused parameter value
  Sub1_out : Outport
  Sub2_out : Outport  Port=2
  Sub3_out : Outport  Port=3
  Sub4_out : Outport  Port=4
  Sub5_out : Outport  Port=5
  Sub6_out : Outport  Port=6
  Sub7_out : Outport  Port=7
  Sub8_out : Outport  Port=8
  Sub9_out : Outport  Port=9
  Sub10_out : Outport  Port=10
  Sub11_out : Outport  Port=11
  Sub12_out : Outport  Port=12
  Sub13_out : Outport  Port=13
  Sub14_out : Outport  Port=14
  wires:
  Sub1/1 -> Bit_Mapping_P1/2(data)
  Sub2/1 -> Bit_Mapping_P2/2(data)
  Bit_Mapping_P1/1(Out1) -> Delay1/1
  Bit_Mapping_P2/1(Out1) -> Delay2/1
  db_sub1_re/1 -> Assert_aft_Mapping/3(sg_sub1_re)
  db_sub1_im/1 -> Assert_aft_Mapping/4(sg_sub1_im)
  Delay1/1 -> Assert_aft_Mapping/1(Sub1), Unbuffer/1
  Delay2/1 -> Assert_aft_Mapping/2(Sub2), Unbuffer1/1
  db_sub2_re/1 -> Assert_aft_Mapping/5(sg_sub2_re)
  db_sub2_im/1 -> Assert_aft_Mapping/6(sg_sub2_im)
  Upsample/1 -> Complex to Real-Imag1/1, Sub1_out/1
  Upsample1/1 -> Sub2_out/1
  Unbuffer/1 -> Upsample/1, Complex to Real-Imag/1
  Complex to Real-Imag/1 -> Scope/1
  Complex to Real-Imag1/1 -> Scope/2
  Unbuffer1/1 -> Upsample1/1, Complex to Real-Imag2/1
  Sub3/1 -> Bit_Mapping_P3/2(data)
  Bit_Mapping_P3/1(Out1) -> Delay3/1
  Delay3/1 -> Sub3_out/1
  Sub4/1 -> Bit_Mapping_P4/2(data)
  Bit_Mapping_P4/1(Out1) -> Delay4/1
  Delay4/1 -> Sub4_out/1
  Sub5/1 -> Bit_Mapping_P5/2(data)
  Bit_Mapping_P5/1(Out1) -> Delay5/1
  Delay5/1 -> Sub5_out/1
  Sub6/1 -> Bit_Mapping_P6/2(data)
  Bit_Mapping_P6/1(Out1) -> Delay6/1
  Delay6/1 -> Sub6_out/1
  Sub7/1 -> Bit_Mapping_P7/2(data)
  Bit_Mapping_P7/1(Out1) -> Delay7/1
  Delay7/1 -> Sub7_out/1
  Sub8/1 -> Bit_Mapping_P8/2(data)
  Bit_Mapping_P8/1(Out1) -> Delay8/1
  Delay8/1 -> Sub8_out/1
  Sub9/1 -> Bit_Mapping_P9/2(data)
  Bit_Mapping_P9/1(Out1) -> Delay9/1
  Delay9/1 -> Sub9_out/1
  Sub10/1 -> Bit_Mapping_P10/2(data)
  Bit_Mapping_P10/1(Out1) -> Delay10/1
  Delay10/1 -> Sub10_out/1
  Sub11/1 -> Bit_Mapping_P11/2(data)
  Bit_Mapping_P11/1(Out1) -> Delay11/1
  Delay11/1 -> Sub11_out/1
  mode/1 -> Bit_Mapping_P2/1(mode), Bit_Mapping_P3/1(mode), Bit_Mapping_P4/1(mode), Bit_Mapping_P5/1(mode), Bit_Mapping_P6/1(mode), Bit_Mapping_P7/1(mode), Bit_Mapping_P8/1(mode), Bit_Mapping_P9/1(mode), Bit_Mapping_P10/1(mode), Bit_Mapping_P11/1(mode), Bit_Mapping_P12/1(mode), Bit_Mapping_P14/1(mode), Bit_Mapping_P13/1(mode), Bit_Mapping_P1/1(mode)
  Sub12/1 -> Bit_Mapping_P12/2(data)
  Bit_Mapping_P12/1(Out1) -> Delay14/1
  Delay14/1 -> Sub12_out/1
  Sub13/1 -> Bit_Mapping_P13/2(data)
  Bit_Mapping_P13/1(Out1) -> Delay12/1
  Delay12/1 -> Sub13_out/1
  Sub14/1 -> Bit_Mapping_P14/2(data)
  Bit_Mapping_P14/1(Out1) -> Delay13/1
  Delay13/1 -> Sub14_out/1
